simulink model "uav_6DOF_ss_v5_1_inner_outer_loop"  (R2022b)
settings: Solver=FixedStepAuto  StartTime=0.0  StopTime=200  FixedStep=1e-2  RelTol=1e-3
InitFcn:
  | drone_init_param
values from neighbouring files (symbols this model uses):
  I_x = 2.24e-3    (= 0.00224)    [uav_6DOF_ss_v5_3_inner_outer_loop_lqr.m]    (also in uav_GA.m; uav_cost_function.m)
  I_y = 2.9e-3    (= 0.0029)    [uav_6DOF_ss_v5_3_inner_outer_loop_lqr.m]    (also in uav_GA.m; uav_cost_function.m)
  I_z = 5.3e-3    (= 0.0053)    [uav_6DOF_ss_v5_3_inner_outer_loop_lqr.m]    (also in uav_GA.m; uav_cost_function.m)
  K_phi = lqi(G_phi,Q_phi,R_phi)    [uav_6DOF_ss_v5_3_inner_outer_loop_lqr.m]    (also in uav_cost_function.m)
  K_theta = lqi(G_theta,Q_theta,R_theta)    [uav_6DOF_ss_v5_3_inner_outer_loop_lqr.m]    (also in uav_cost_function.m)
  K_x = lqi(G_x,Q_x,R_x)    [uav_6DOF_ss_v5_3_inner_outer_loop_lqr.m]    (also in uav_cost_function.m)
  K_y = lqi(G_y,Q_y,R_y)    [uav_6DOF_ss_v5_3_inner_outer_loop_lqr.m]    (also in uav_cost_function.m)
  K_yaw = lqi(G_yaw,Q_yaw,R_yaw)    [uav_6DOF_ss_v5_3_inner_outer_loop_lqr.m]    (also in uav_cost_function.m)
  K_z = lqi(G_z,Q_z,R_z)    [uav_6DOF_ss_v5_3_inner_outer_loop_lqr.m]    (also in uav_cost_function.m)
  m = 0.46    [uav_6DOF_ss_v5_3_inner_outer_loop_lqr.m]    (also in uav_GA.m; uav_cost_function.m)
settings Model: Creator=Ali Tahir  LastModifiedBy=Ali Tahir

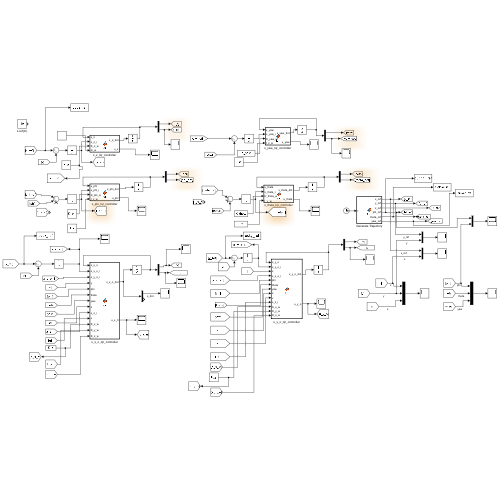
[thumbnail: Simulink's stored preview of the top-level diagram]
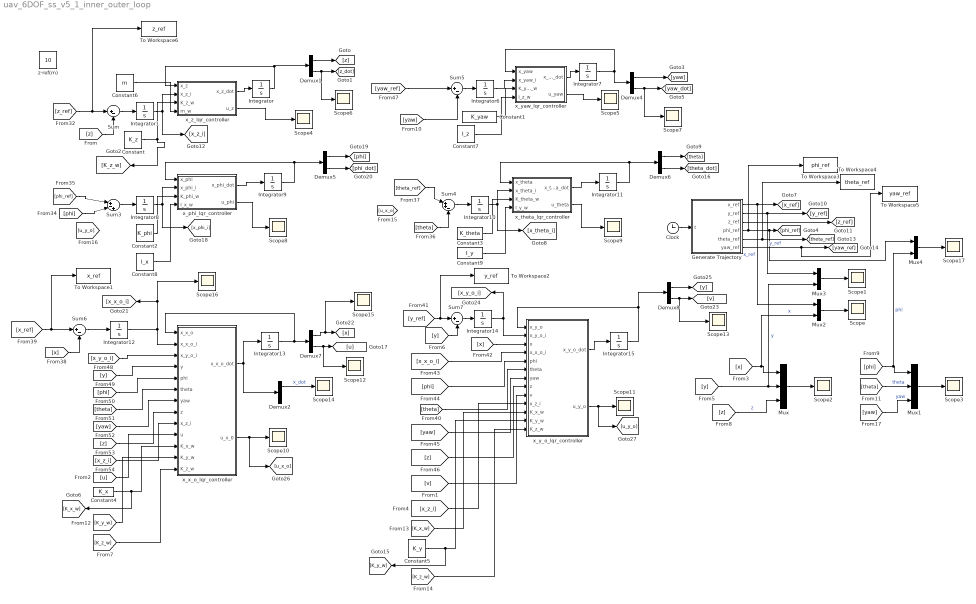
== system uav_6DOF_ss_v5_1_inner_outer_loop ==
  Clock : Clock
  Constant : Constant  Value=K_z
  Constant1 : Constant  Value=K_yaw
  Constant2 : Constant  Value=K_phi
  Constant3 : Constant  Value=K_theta
  Constant4 : Constant  Value=K_x
  Constant5 : Constant  Value=K_y
  Constant6 : Constant  Value=m
  Constant7 : Constant  Value=I_z
  Constant8 : Constant  Value=I_x
  Constant9 : Constant  Value=I_y
  Demux{1..2,4..8} (7 alike) : Demux  Outputs=2
  Generate Trajectory : MATLAB Function  TreatAsAtomicUnit=on
  Integrator{,7,9,11,13,15} (6 alike) : Integrator  InitialCondition=[0;0]
  Integrator{1,6,8,10,12,14} (6 alike) : Integrator
  Mux : Mux  Inputs=3
  Mux1 : Mux  Inputs=3
  Mux2 : Mux  Inputs=2
  Mux3 : Mux  Inputs=2
  Mux4 : Mux  Inputs=2
  Scope{,1..17} (18 alike) : Scope
  Sum{,5..7} (4 alike) : Sum  Inputs=|+-
  Sum3 : Sum  Inputs=|+-+
  Sum4 : Sum  Inputs=|++-
  To Workspace1 : ToWorkspace  VariableName=x_ref  SampleTime=-1
  To Workspace2 : ToWorkspace  VariableName=y_ref  SampleTime=-1
  To Workspace3 : ToWorkspace  VariableName=phi_ref  SampleTime=-1
  To Workspace4 : ToWorkspace  VariableName=theta_ref  SampleTime=-1
  To Workspace5 : ToWorkspace  VariableName=yaw_ref  SampleTime=-1
  To Workspace6 : ToWorkspace  VariableName=z_ref  SampleTime=-1
  x_phi_lqr_controller : MATLAB Function  TreatAsAtomicUnit=on
  x_theta_lqr_controller : MATLAB Function  TreatAsAtomicUnit=on
  x_x_o_lqr_controller : MATLAB Function  TreatAsAtomicUnit=on
  x_y_o_lqr_controller : MATLAB Function  TreatAsAtomicUnit=on
  x_yaw_lqr_controller : MATLAB Function  TreatAsAtomicUnit=on
  x_z_lqr_controller : MATLAB Function  TreatAsAtomicUnit=on
  z-ref(m) : Constant  Value=10
  wires:
  [z] -> Sum/2
  Sum/1 -> Integrator1/1
  Integrator1/1 -> [x_z_i], x_z_lqr_controller/2(x_z_i)
  [yaw] -> Sum5/2
  [yaw_ref] -> Sum5/1
  Sum5/1 -> Integrator6/1
  Integrator6/1 -> x_yaw_lqr_controller/2(x_yaw_i)
  x_z_lqr_controller/1(x_z_dot) -> Integrator/1
  Integrator/1 -> Demux1/1, x_z_lqr_controller/1(x_z)
  Demux1/1 -> [z]
  Demux1/2 -> Scope6/1, [z_dot]
  Integrator7/1 -> Demux4/1, x_yaw_lqr_controller/1(x_yaw)
  Demux4/1 -> [yaw]
  Demux4/2 -> Scope7/1, [yaw_dot]
  x_yaw_lqr_controller/1(x_yaw_dot) -> Integrator7/1
  [x] -> Mux2/2, Mux/1  "x"
  [z] -> Mux/3  "z"
  Mux/1 -> Scope2/1
  [yaw] -> Mux1/3  "yaw"
  [phi] -> Mux4/2, Mux1/1  "phi"
  [theta] -> Mux1/2  "theta"
  Mux1/1 -> Scope3/1
  x_z_lqr_controller/2(u_z) -> Scope4/1
  x_yaw_lqr_controller/2(u_yaw) -> Scope5/1
  Clock/1 -> Generate Trajectory/1(t)
  Generate Trajectory/2(y_ref) -> Mux3/1, [y_ref]  "y_ref"
  Generate Trajectory/3(z_ref) -> [z_ref]
  [z_ref] -> To Workspace6/1, Sum/1
  Integrator8/1 -> [x_phi_i], x_phi_lqr_controller/2(x_phi_i)
  [phi_ref] -> Sum3/1
  Sum3/1 -> Integrator8/1
  [phi] -> Sum3/2
  x_phi_lqr_controller/1(x_phi_dot) -> Integrator9/1
  x_phi_lqr_controller/2(u_phi) -> Scope8/1
  Integrator9/1 -> Demux5/1, x_phi_lqr_controller/1(x_phi)
  Demux5/1 -> [phi]
  Demux5/2 -> [phi_dot]
  Demux6/2 -> [theta_dot]
  x_theta_lqr_controller/1(x_theta_dot) -> Integrator11/1
  x_theta_lqr_controller/2(u_theta) -> Scope9/1
  Sum4/1 -> Integrator10/1
  Integrator10/1 -> [x_theta_i], x_theta_lqr_controller/2(x_theta_i)
  Integrator11/1 -> Demux6/1, x_theta_lqr_controller/1(x_theta)
  [theta_ref] -> Sum4/1
  Demux6/1 -> [theta]
  Demux7/1 -> Scope15/1, [x]
  Integrator13/1 -> x_x_o_lqr_controller/1(x_x_o), Demux7/1
  [x_ref] -> To Workspace1/1, Sum6/1
  Sum6/1 -> Integrator12/1
  Integrator12/1 -> x_x_o_lqr_controller/2(x_x_o_i), Scope16/1, [x_x_o_i]
  Demux7/2 -> Scope12/1, [u]
  [x] -> Sum6/2
  x_x_o_lqr_controller/2(u_x_0) -> [u_x_o], Scope10/1
  x_x_o_lqr_controller/1(x_x_o_dot) -> Integrator13/1, Demux2/1
  Demux8/1 -> [y]
  Integrator15/1 -> Demux8/1, x_y_o_lqr_controller/1(x_y_o)
  [y_ref] -> To Workspace2/1, Sum7/1
  Sum7/1 -> Integrator14/1
  Integrator14/1 -> x_y_o_lqr_controller/2(x_y_o_i), [x_y_o_i]
  Demux8/2 -> Scope13/1, [v]
  [theta] -> x_y_o_lqr_controller/6(theta)
  x_y_o_lqr_controller/2(u_y_o) -> [u_y_o], Scope11/1
  x_y_o_lqr_controller/1(x_y_o_dot) -> Integrator15/1
  [x] -> x_y_o_lqr_controller/3(x)
  [x_x_o_i] -> x_y_o_lqr_controller/4(x_x_o_i)
  [phi] -> x_y_o_lqr_controller/5(phi)
  [yaw] -> x_y_o_lqr_controller/7(yaw)
  [z] -> x_y_o_lqr_controller/8(z)
  Generate Trajectory/4(phi_ref) -> To Workspace3/1, Mux4/1, [phi_ref]
  Generate Trajectory/5(theta_ref) -> To Workspace4/1, [theta_ref]
  Generate Trajectory/6(yaw_ref) -> To Workspace5/1, [yaw_ref]
  [x_y_o_i] -> x_x_o_lqr_controller/3(x_y_o_i)
  [y] -> x_x_o_lqr_controller/4(y)
  [phi] -> x_x_o_lqr_controller/5(phi)
  [theta] -> x_x_o_lqr_controller/6(theta)
  [yaw] -> x_x_o_lqr_controller/7(yaw)
  [z] -> x_x_o_lqr_controller/8(z)
  [x_z_i] -> x_x_o_lqr_controller/9(x_z_i)
  [v] -> x_y_o_lqr_controller/9(v)
  [u] -> x_x_o_lqr_controller/10(u)
  [x_z_i] -> x_y_o_lqr_controller/10(x_z_i)
  Mux2/1 -> Scope/1
  Generate Trajectory/1(x_ref) -> [x_ref], Mux2/1  "x_ref"
  Mux3/1 -> Scope1/1
  [y] -> Mux3/2, Mux/2  "y"
  [y] -> Sum7/2
  Constant/1 -> [K_z_w], x_z_lqr_controller/3(K_z_w)
  Constant1/1 -> x_yaw_lqr_controller/3(K_yaw_w)
  Constant2/1 -> x_phi_lqr_controller/3(K_phi_w)
  Constant3/1 -> x_theta_lqr_controller/3(K_theta_w)
  [K_z_w] -> x_x_o_lqr_controller/13(K_z_w)
  Constant4/1 -> [K_x_w], x_x_o_lqr_controller/11(K_x_w)
  [K_y_w] -> x_x_o_lqr_controller/12(K_y_w)
  [K_x_w] -> x_y_o_lqr_controller/11(K_x_w)
  [K_z_w] -> x_y_o_lqr_controller/13(K_z_w)
  Constant5/1 -> [K_y_w], x_y_o_lqr_controller/12(K_y_w)
  Constant6/1 -> x_z_lqr_controller/4(m_w)
  Constant7/1 -> x_yaw_lqr_controller/4(I_z_w)
  Constant8/1 -> x_phi_lqr_controller/4(I_x_w)
  Constant9/1 -> x_theta_lqr_controller/4(I_y_w)
  [theta] -> Sum4/3
  Demux2/1 -> Scope14/1  "x_dot"
  Mux4/1 -> Scope17/1

== matlab function uav_6DOF_ss_v5_1_inner_outer_loop/x_y_o_lqr_controller ==
  data: x_y_o input; x_y_o_dot output; x_y_o_i input; u_y_o output; x input; x_x_o_i input; phi input; theta input; yaw input; z input; v input; x_z_i input; K_x_w input; K_y_w input; K_z_w input
function [x_y_o_dot, u_y_o] = lqr(x_y_o, x_y_o_i, x, x_x_o_i, phi, theta, yaw, z, v, x_z_i, K_x_w, K_y_w, K_z_w)
g = 9.81;          % gravity                       (m/s^2)

% Ky_o = [-0.2453 -0.2259];
% Ky_o_i = 0.1000;
% 
% Kz1 = 2.2026;
% Kz2 = -1.0000;
% 
% Kx_o_1 = 0.2453;
% Kx_o_i = -0.1000;
K_x_w = K_x_w';
K_y_w = K_y_w';
K_z_w = K_z_w';

Ky_o = K_y_w(1,1:2);
Ky_o_i = K_y_w(1,3);

Kz1 = K_z_w(1,1);
Kz2 = K_z_w(1,3);

Kx_o_1 = K_x_w(1,1);
Kx_o_i = K_x_w(1,3);

A = zeros(2,2);
B = zeros(2,1);

A(1,2) = 1;
B(2,1) = -g;

a = ((sin(phi)*cos(theta)) * ((-Kx_o_1 * x) - (Kx_o_i * x_x_o_i)));
b = (((sin(phi)*sin(theta)*sin(yaw))+(cos(phi)*cos(yaw))) * ((-Ky_o(1,1)*x_y_o(1,1)) - (Ky_o_i * x_y_o_i)));
c = (((sin(phi)*sin(theta)*cos(yaw))-(cos(phi)*sin(yaw))) * ((-Kz1*z) - (Kz2* x_z_i)));

u_y_o = (a+b+c) - (Ky_o(1,2) * v) - (phi);

x_y_o_dot = A * x_y_o + B * u_y_o;

end

== matlab function uav_6DOF_ss_v5_1_inner_outer_loop/Generate Trajectory ==
  settings: updateMethod=DISCRETE  sampleTime=0.01
  data: t input; x_ref output; y_ref output; z_ref output; phi_ref output; theta_ref output; yaw_ref output
function [x_ref, y_ref, z_ref, phi_ref, theta_ref, yaw_ref] = fcn(t)


% GA-LQR study reference
%     x_ref = 0;
%     y_ref = 0;
%     z_ref = 0;

    % Step response
%     if t >= 0 && t < 5        
%         z_ref = 0;
%         x_ref = 0;
%         y_ref = 0;
%         phi_ref = 0;
%         theta_ref = 0;
%         yaw_ref = 0;
%     
%     elseif t >= 5 && t < 15
%         z_ref = 0;
%         x_ref = 1;%1       
%         y_ref = 0;  
%         phi_ref = 0;
%         theta_ref = 0;
%         yaw_ref = 0;
%     
%     elseif t >= 15 && t < 25
%         z_ref = 0;
%         y_ref = 1;
%         x_ref = 0;
%         phi_ref = 0;
%         theta_ref = 0;
%         yaw_ref = 0;
%     
%     elseif t >= 25 && t < 35
%         z_ref = 1;
%         y_ref = 0;
%         x_ref = 0;
%         phi_ref = 0;
%         theta_ref = 0;
%         yaw_ref = 0;
%     
%     elseif t >= 35 && t < 45
%         z_ref = 0;        
%         y_ref = 0;
%         x_ref = 0;
%         phi_ref = 0.2;
%         theta_ref = 0;
%         yaw_ref = 0;
%     
%     elseif t>= 45 && t <= 55
%         z_ref = 0;
%          y_ref =0;
%          x_ref = 0;
%          phi_ref = 0;
%         theta_ref = 0.2;
%         yaw_ref = 0;
%     else
%          z_ref = 0;
%          y_ref =0;
%          x_ref = 0;
%          phi_ref = 0;
%         theta_ref = 0;
%         yaw_ref = 0.2;
%     end
 


    %%3D trajectory
    phi_ref = 0;
    theta_ref = 0;
    yaw_ref = 0;
    
    if t >= 0 && t < 10        
        z_ref = 0;
        x_ref = 0;
        y_ref = 0;
    
    elseif t >= 10 && t < 60
        z_ref = 0.75;
        x_ref = (t/50) - 0.2;%1       
        y_ref = 0;        
    
    elseif t >= 60 && t < 100
        z_ref = 1.25;
        y_ref = (-0.025*t)+1.5;
         x_ref = 1.5;
    
    elseif t >= 100 && t < 150
        z_ref = 0.75;
         y_ref = -1;
          x_ref = 1;
    
    elseif t >= 150 && t < 180
        z_ref = 1.25;
        %y_ref=-1
        y_ref = 0.02*t -4;
        x_ref = (-0.0333*t +6);%0
    
    else %t >= 180 && t <= 200
        z_ref = 0.75;
         y_ref = 0.02*t -4;
         x_ref = -1;
    end
 
  
% GA-FPID study
% if t>= 0 && t < 25
%     x_ref = 0;
%     y_ref = 0;
%     z_ref = t/ 16.667;%1.5;
%     
%     phi_ref = 0;
%     theta_ref = 0;
%     yaw_ref = 0;
% 
% elseif t>= 25 && t < 50
%     x_ref = 3;
%     y_ref = 2;
%     z_ref = 1.5;
%     
%     phi_ref = 0;
%     theta_ref = 0;
%     yaw_ref = 0;
% 
% elseif t>= 50 && t < 75
%     x_ref = 5;
%     y_ref = 2;
%     z_ref = 1.5;
%     
%     phi_ref = 0;
%     theta_ref = 0;
%     yaw_ref = 0;
% 
% elseif t>= 75 && t < 100
%     x_ref = 4 + (cos(t / 4));
%     y_ref = 2 + sin(t / 4);
%     z_ref = 1.5;
%     
%     phi_ref = 0;
%     theta_ref = 0;
%     yaw_ref = 0;
% 
% elseif t>= 100 && t < 125  
%     x_ref = 4 + (cos(t/4));
%     y_ref = 2 + (sin(2 * (t/4))/2);
%     z_ref = 1.5;
%     
%     phi_ref = 0;
%     theta_ref = 0;
%     yaw_ref = 0;
% else
%     x_ref = 5;
%     y_ref = 2;
%     z_ref = 1;
%     
%     phi_ref = 0;
%     theta_ref = 0;
%     yaw_ref = 0;
% end

end

== matlab function uav_6DOF_ss_v5_1_inner_outer_loop/x_z_lqr_controller ==
  data: x_z input; x_z_dot output; x_z_i input; u_z output; K_z_w input; m_w input
function [x_z_dot, u_z] = lqr(x_z, x_z_i, K_z_w, m_w)
m = m_w;

%def 1-1-1
% Kz = [ 2.2026    1.5925];
% K1_z = -1.0000;

K_z_w = K_z_w';
Kz = K_z_w(1,1:2);
K1_z = K_z_w(1,3);

u_z = -Kz * x_z - K1_z * x_z_i;

A = zeros(2,2);
B = zeros(2,1);

A(1,2) = 1;
B(2,1) = 1/m;

x_z_dot = A * x_z + B * u_z;

end

== matlab function uav_6DOF_ss_v5_1_inner_outer_loop/x_phi_lqr_controller ==
  data: x_phi input; x_phi_dot output; x_phi_i input; u_phi output; K_phi_w input; I_x_w input
function [x_phi_dot, u_phi] = lqr(x_phi, x_phi_i, K_phi_w, I_x_w)

%def 1-1-1
I_x = I_x_w;    % moment of inertia of uav      (kg.m^2)
    
% Kphi = [1.1654 0.2251];
% K1_phi = -2.7386;

K_phi_w = K_phi_w';
Kphi = K_phi_w(1,1:2);
K1_phi = K_phi_w(1,3);

u_phi = -Kphi * x_phi - K1_phi * x_phi_i;

A = zeros(2,2);
B = zeros(2,1);

A(1,2) = 1;
B(2,1) = 1/I_x;

x_phi_dot = A * x_phi + B * u_phi;

end

== matlab function uav_6DOF_ss_v5_1_inner_outer_loop/x_theta_lqr_controller ==
  data: x_theta input; x_theta_dot output; x_theta_i input; u_theta output; K_theta_w input; I_y_w input
function [x_theta_dot, u_theta] = lqr(x_theta, x_theta_i, K_theta_w, I_y_w)

I_y = I_y_w;

K_theta_w = K_theta_w';
Ktheta = K_theta_w(1,1:2);
Ktheta_i = K_theta_w(1,3);

u_theta = -Ktheta * x_theta - Ktheta_i * x_theta_i;

A = zeros(2,2);
B = zeros(2,1);

A(1,2) = 1;
B(2,1) = 1/I_y;

x_theta_dot = A * x_theta + B * u_theta;

end

== matlab function uav_6DOF_ss_v5_1_inner_outer_loop/x_yaw_lqr_controller ==
  data: x_yaw input; x_yaw_dot output; x_yaw_i input; u_yaw output; K_yaw_w input; I_z_w input
function [x_yaw_dot, u_yaw] = lqr(x_yaw, x_yaw_i, K_yaw_w, I_z_w)

I_z = I_z_w;

A = zeros(2,2);
B = zeros(2,1);

A(1,2) = 1;
B(2,1) = 1 / I_z;

% Kyaw = [3.9387    1.0991];
% Kyaw_i = -3.8730;

K_yaw_w = K_yaw_w';
Kyaw = K_yaw_w(1,1:2);
Kyaw_i = K_yaw_w(1,3);

u_yaw = -Kyaw * x_yaw - Kyaw_i * x_yaw_i;

x_yaw_dot = A * x_yaw + B * u_yaw;

end

== matlab function uav_6DOF_ss_v5_1_inner_outer_loop/x_x_o_lqr_controller ==
  data: x_x_o input; x_x_o_dot output; x_x_o_i input; u_x_0 output; x_y_o_i input; y input; phi input; theta input; yaw input; z input; x_z_i input; u input; K_x_w input; K_y_w input; K_z_w input
function [x_x_o_dot, u_x_0] = lqr(x_x_o, x_x_o_i, x_y_o_i, y, phi, theta, yaw, z, x_z_i, u, K_x_w, K_y_w, K_z_w)

g = 9.81;          % gravity                       (m/s^2)

% Kx_o = [0.2453    0.2259];
% Kx_o_i =  -0.1000;
% 
% Ky_o_1 = -0.2453;
% Ky_o_i = 0.1000;
% 
% Kz1 = 2.2026;
% Kz_i = -1.0000;

K_x_w = K_x_w';
K_y_w = K_y_w';
K_z_w = K_z_w';

Kx_o = K_x_w(1,1:2);
Kx_o_i = K_x_w(1,3);

Ky_o_1 = K_y_w(1,1);
Ky_o_i = K_y_w(1,3);

Kz1 = K_z_w(1,1);
Kz_i = K_z_w(1,3);

A = zeros(2,2);
B = zeros(2,1);

A(1,2) = 1;
B(2,1) = g;

a = ((cos(theta)*cos(phi)) * (-Kx_o(1,1)*x_x_o(1,1) - (Kx_o_i * x_x_o_i)));
b = (((cos(phi)*sin(theta)*sin(yaw))-(sin(phi)*cos(yaw))) * ((-Ky_o_1*y) - (Ky_o_i * x_y_o_i)));
c = (((cos(phi)*sin(theta)*cos(yaw))+(sin(phi)*sin(yaw))) * ((-Kz1*z) - (Kz_i*x_z_i)));

u_x_0 = (a+b+c) - (Kx_o(1,2) * u) - (theta);

x_x_o_dot = A * x_x_o + B * u_x_0;

end
